simulink model "dds_osc_test"  (Simulink 7.0)
settings: Solver=VariableStepDiscrete  StartTime=0.0  StopTime=1000  RelTol=1e-3
libraries: xbsIndex_r4 x5, casper_library x2
settings Model: Creator=User  LastModifiedBy=User
settings DebuggingCC: SaveWithDisabledLinksMsg=none  SaveWithParameterizedLinksMsg=none

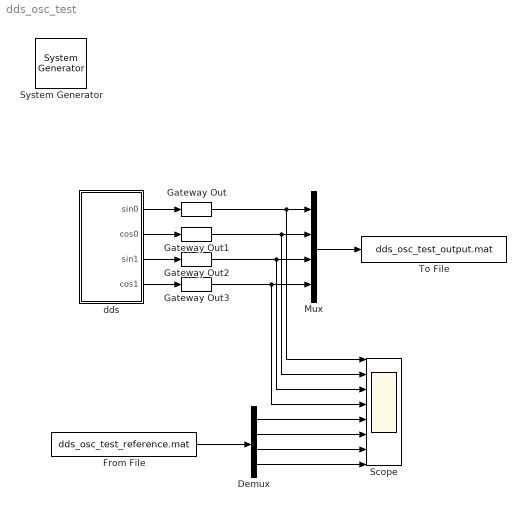
== system dds_osc_test ==
  " System Generator" : xbsIndex_r4/ System Generator  Tag=genX  SystemSampleTime=-1  xilinxfamily=Virtex4  part=xc4vsx35  speed=-10  package=ff668  synthesis_tool=XST  clock_wrapper=Clock Enables  directory=./netlist  testbench=off  simulink_period=1  sysclk_period=100  dcm_input_clock_period=100  incr_netlist=off  trim_vbits=Everywhere in SubSystem  dbl_ovrd=According to Block Masks  core_generation=According to Block Masks  run_coregen=off  deprecated_control=off  eval_field=0  block_type=sysgen
      settings: block_version=10.1.1
  Demux : Demux
  From File : FromFile  FileName=dds_osc_test_reference.mat  SampleTime=1
  Gateway Out{,1..3} (4 alike) : xbsIndex_r4/Gateway Out  hdl_port=on  timing_constraint=None  locs_specified=off  LOCs={}  block_type=gatewayout
      settings: infoedit="Gateway out block.  Converts Xilinx fixed point inputs into ouputs of type Simulink integer, double, or fixed point.<P><P>Hardware notes:  In hardware these blocks become top level output ports or are discarded, depending on how they are configured."  block_version=10.1.1
  Mux : Mux
  Scope : Scope  NumInputPorts=8
      settings: YMin=-5~-5~-5~-5~-5~-5~-5~-5  YMax=5~5~5~5~5~5~5~5
  To File : ToFile  Filename=dds_osc_test_output.mat  MatrixName=output
  dds : Subsystem  AncestorBlock=casper_library/Downconverter/dds  mask(dds){freq_div=4, freq=1, num_lo=2, n_bits=8, latency=3}
      mask prompts: freq_div "Frequency divisions (M)"; freq "Frequency (? / M*2pi)"; num_lo "Parallel LOs"; n_bits "Bit Width"
      mask help:
      | Generates P channels of sin and cos data for mixing
      | with input data in a DDC. To generate frequency
      | N/M(Fc x P) (where Fc is the clock rate)
      | M = "Frequency Divisions", N = "Frequency",
      | Parallel LOs = P
      mask init:
      | dds_init(gcb, ...
      |     'freq_div', freq_div, ...
      |     'freq', freq, ...
      |     'num_lo', num_lo, ...
      |     'n_bits', n_bits, ...
      |     'latency', latency);
      settings: AttributesFormatString=lo at -1/4
      mask Help: eval('xlWeb([getenv(''MLIB_ROOT''), ''\doc\htmlblocks\sp_dds\sp_dds.html''])')
  wires:
  dds/1(sin0) -> Gateway Out/1
  dds/2(cos0) -> Gateway Out1/1
  dds/3(sin1) -> Gateway Out2/1
  dds/4(cos1) -> Gateway Out3/1
  Gateway Out/1 -> Mux/1, Scope/1
  Gateway Out1/1 -> Mux/2, Scope/2
  Gateway Out2/1 -> Mux/3, Scope/3
  Gateway Out3/1 -> Mux/4, Scope/4
  Mux/1 -> To File/1
  From File/1 -> Demux/1
  Demux/1 -> Scope/5
  Demux/2 -> Scope/6
  Demux/3 -> Scope/7
  Demux/4 -> Scope/8

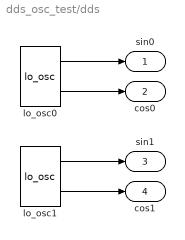
== system dds_osc_test/dds ==
  lo_osc0 : casper_library/Downconverter/lo_osc  SystemSampleTime=-1  n_bits=8  counter_step=2  counter_start=0  counter_width=2  latency=3
  lo_osc1 : casper_library/Downconverter/lo_osc  SystemSampleTime=-1  n_bits=8  counter_step=2  counter_start=1  counter_width=2  latency=3
      link override counter: start_count=counter_start*4  cnt_by_val=counter_step*4  n_bits=counter_width+2
  sin0 : Outport  OutDataType=sfix(16)  OutScaling=2^0
  cos0 : Outport  Port=2  OutDataType=sfix(16)  OutScaling=2^0
  sin1 : Outport  Port=3  OutDataType=sfix(16)  OutScaling=2^0
  cos1 : Outport  Port=4  OutDataType=sfix(16)  OutScaling=2^0
  wires:
  lo_osc1/2 -> cos1/1
  lo_osc1/1 -> sin1/1
  lo_osc0/2 -> cos0/1
  lo_osc0/1 -> sin0/1
